simulink model "Samuno_Experimental"  (R2024b)
settings: Solver=ode4  StartTime=0.0  StopTime=Dur  FixedStep=simulation_ts  RelTol=1e-3  AbsTol=1e-3
InitFcn:
  | run("init_parts.m");
model workspace (MAT data in the model file):
  Control_Range_Lim = 0.2086
  D_Heading = 0
  I_Heading = 0
  P_Heading = 1
  control_ts = 0.4
  kd_pitch = 0
  kd_roll = 0.1
  kp_pitch = 4
  kp_roll = 4
  random_velocity = 0.72
  switch_val = 0.1032
values from neighbouring files (symbols this model uses):
  Nose = evalin('base', 'Nose')    [createSimulinkGUI.m]
  xCOB = xSliderCOB.Value    [createSimulinkGUI.m]
  zCOB = ySliderCOB.Value    [createSimulinkGUI.m]
undefined symbols (not defined in the file or in its folder): Caudal, colors, Force_Scale, gravity, Mid_Body, Mid_Fins, noise_mean, noise_sample_time, noise_var, Pect, Pedunc, TotalMass, X, Y, Z
libraries: nesl_utility x84, sm_lib x53
(part 3 of 3)

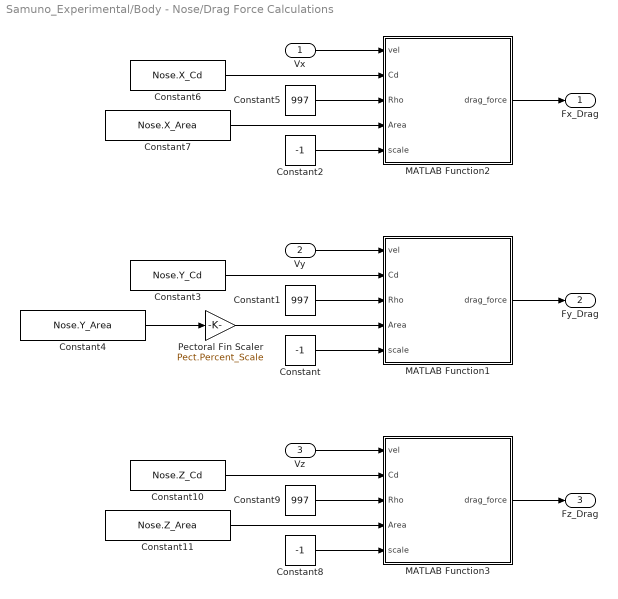
== system Samuno_Experimental/Body - Nose/Drag Force Calculations ==
  Vx : Inport
  Vy : Inport  Port=2
  Vz : Inport  Port=3
  Constant : Constant  Value=-1
  Constant1 : Constant  Value=997
  Constant10 : Constant  Value=Nose.Z_Cd
  Constant11 : Constant  Value=Nose.Z_Area
  Constant2 : Constant  Value=-1
  Constant3 : Constant  Value=Nose.Y_Cd
  Constant4 : Constant  Value=Nose.Y_Area
  Constant5 : Constant  Value=997
  Constant6 : Constant  Value=Nose.X_Cd
  Constant7 : Constant  Value=Nose.X_Area
  Constant8 : Constant  Value=-1
  Constant9 : Constant  Value=997
  MATLAB Function1 : MATLAB Function  TreatAsAtomicUnit=on
  MATLAB Function2 : MATLAB Function  TreatAsAtomicUnit=on
  MATLAB Function3 : MATLAB Function  TreatAsAtomicUnit=on
  Pectoral Fin Scaler : Gain  Gain=Pect.Percent_Scale
  Fx_Drag : Outport
  Fy_Drag : Outport  Port=2
  Fz_Drag : Outport  Port=3
  wires:
  Constant1/1 -> MATLAB Function1/3(Rho)
  MATLAB Function1/1(drag_force) -> Fy_Drag/1
  Constant4/1 -> Pectoral Fin Scaler/1
  Constant/1 -> MATLAB Function1/5(scale)
  Vy/1 -> MATLAB Function1/1(vel)
  Constant3/1 -> MATLAB Function1/2(Cd)
  Constant6/1 -> MATLAB Function2/2(Cd)
  Constant2/1 -> MATLAB Function2/5(scale)
  Constant7/1 -> MATLAB Function2/4(Area)
  Vx/1 -> MATLAB Function2/1(vel)
  MATLAB Function2/1(drag_force) -> Fx_Drag/1
  Constant5/1 -> MATLAB Function2/3(Rho)
  MATLAB Function3/1(drag_force) -> Fz_Drag/1
  Constant8/1 -> MATLAB Function3/5(scale)
  Constant11/1 -> MATLAB Function3/4(Area)
  Constant10/1 -> MATLAB Function3/2(Cd)
  Vz/1 -> MATLAB Function3/1(vel)
  Constant9/1 -> MATLAB Function3/3(Rho)
  Pectoral Fin Scaler/1 -> MATLAB Function1/4(Area)

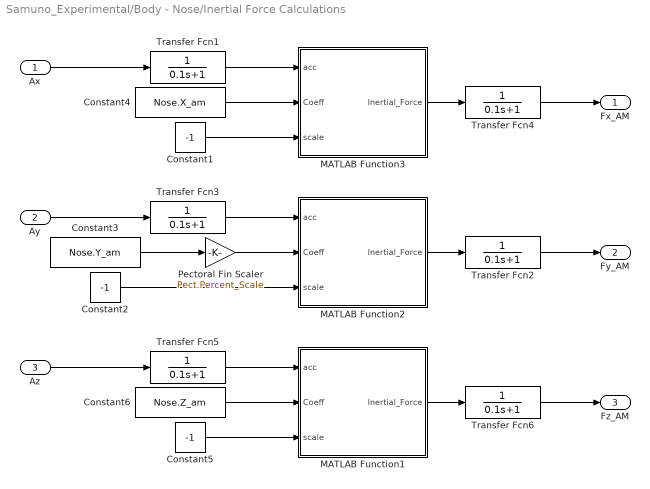
== system Samuno_Experimental/Body - Nose/Inertial Force Calculations ==
  Ax : Inport
  Ay : Inport  Port=2
  Az : Inport  Port=3
  Constant1 : Constant  Value=-1
  Constant2 : Constant  Value=-1
  Constant3 : Constant  Value=Nose.Y_am
  Constant4 : Constant  Value=Nose.X_am
  Constant5 : Constant  Value=-1
  Constant6 : Constant  Value=Nose.Z_am
  MATLAB Function1 : MATLAB Function  TreatAsAtomicUnit=on
  MATLAB Function2 : MATLAB Function  TreatAsAtomicUnit=on
  MATLAB Function3 : MATLAB Function  TreatAsAtomicUnit=on
  Pectoral Fin Scaler : Gain  Gain=Pect.Percent_Scale
  Transfer Fcn{1..6} (6 alike) : TransferFcn  Denominator=[0.1 1]
  Fx_AM : Outport
  Fy_AM : Outport  Port=2
  Fz_AM : Outport  Port=3
  wires:
  Ax/1 -> Transfer Fcn1/1
  Constant1/1 -> MATLAB Function3/3(scale)
  Transfer Fcn1/1 -> MATLAB Function3/1(acc)
  Constant4/1 -> MATLAB Function3/2(Coeff)
  Transfer Fcn4/1 -> Fx_AM/1
  MATLAB Function3/1(Inertial_Force) -> Transfer Fcn4/1
  Ay/1 -> Transfer Fcn3/1
  Constant2/1 -> MATLAB Function2/3(scale)
  Transfer Fcn3/1 -> MATLAB Function2/1(acc)
  Constant3/1 -> Pectoral Fin Scaler/1
  Transfer Fcn2/1 -> Fy_AM/1
  MATLAB Function2/1(Inertial_Force) -> Transfer Fcn2/1
  Az/1 -> Transfer Fcn5/1
  Constant5/1 -> MATLAB Function1/3(scale)
  Transfer Fcn5/1 -> MATLAB Function1/1(acc)
  Constant6/1 -> MATLAB Function1/2(Coeff)
  Transfer Fcn6/1 -> Fz_AM/1
  MATLAB Function1/1(Inertial_Force) -> Transfer Fcn6/1
  Pectoral Fin Scaler/1 -> MATLAB Function2/2(Coeff)

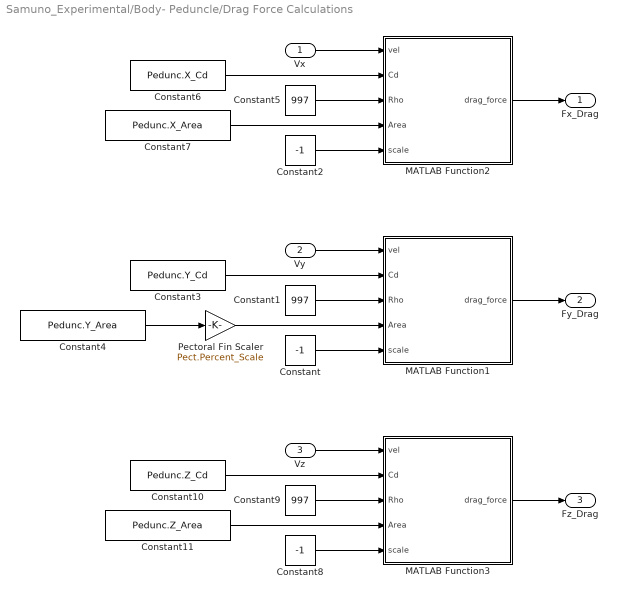
== system Samuno_Experimental/Body- Peduncle/Drag Force Calculations ==
  Vx : Inport
  Vy : Inport  Port=2
  Vz : Inport  Port=3
  Constant : Constant  Value=-1
  Constant1 : Constant  Value=997
  Constant10 : Constant  Value=Pedunc.Z_Cd
  Constant11 : Constant  Value=Pedunc.Z_Area
  Constant2 : Constant  Value=-1
  Constant3 : Constant  Value=Pedunc.Y_Cd
  Constant4 : Constant  Value=Pedunc.Y_Area
  Constant5 : Constant  Value=997
  Constant6 : Constant  Value=Pedunc.X_Cd
  Constant7 : Constant  Value=Pedunc.X_Area
  Constant8 : Constant  Value=-1
  Constant9 : Constant  Value=997
  MATLAB Function1 : MATLAB Function  TreatAsAtomicUnit=on
  MATLAB Function2 : MATLAB Function  TreatAsAtomicUnit=on
  MATLAB Function3 : MATLAB Function  TreatAsAtomicUnit=on
  Pectoral Fin Scaler : Gain  Gain=Pect.Percent_Scale
  Fx_Drag : Outport
  Fy_Drag : Outport  Port=2
  Fz_Drag : Outport  Port=3
  wires:
  Constant1/1 -> MATLAB Function1/3(Rho)
  MATLAB Function1/1(drag_force) -> Fy_Drag/1
  Constant4/1 -> Pectoral Fin Scaler/1
  Constant/1 -> MATLAB Function1/5(scale)
  Vy/1 -> MATLAB Function1/1(vel)
  Constant3/1 -> MATLAB Function1/2(Cd)
  Constant6/1 -> MATLAB Function2/2(Cd)
  Constant2/1 -> MATLAB Function2/5(scale)
  Constant7/1 -> MATLAB Function2/4(Area)
  Vx/1 -> MATLAB Function2/1(vel)
  MATLAB Function2/1(drag_force) -> Fx_Drag/1
  Constant5/1 -> MATLAB Function2/3(Rho)
  MATLAB Function3/1(drag_force) -> Fz_Drag/1
  Constant8/1 -> MATLAB Function3/5(scale)
  Constant11/1 -> MATLAB Function3/4(Area)
  Constant10/1 -> MATLAB Function3/2(Cd)
  Vz/1 -> MATLAB Function3/1(vel)
  Constant9/1 -> MATLAB Function3/3(Rho)
  Pectoral Fin Scaler/1 -> MATLAB Function1/4(Area)

== system Samuno_Experimental/Body- Peduncle/Inertial Force Calculations ==
  Ax : Inport
  Ay : Inport  Port=2
  Az : Inport  Port=3
  Constant1 : Constant  Value=-1
  Constant2 : Constant  Value=-1
  Constant3 : Constant  Value=Pedunc.Y_am
  Constant4 : Constant  Value=Pedunc.X_am
  Constant5 : Constant  Value=-1
  Constant6 : Constant  Value=Pedunc.Z_am
  MATLAB Function1 : MATLAB Function  TreatAsAtomicUnit=on
  MATLAB Function2 : MATLAB Function  TreatAsAtomicUnit=on
  MATLAB Function3 : MATLAB Function  TreatAsAtomicUnit=on
  Pectoral Fin Scaler : Gain  Gain=Pect.Percent_Scale
  Transfer Fcn1 : TransferFcn  Numerator=1.5  Denominator=[0.005 1]
  Transfer Fcn2 : TransferFcn  Numerator=1.5  Denominator=[0.005 1]
  Transfer Fcn3 : TransferFcn  Numerator=1.5  Denominator=[0.005 1]
  Fx_AM : Outport
  Fy_AM : Outport  Port=2
  Fz_AM : Outport  Port=3
  wires:
  Constant1/1 -> MATLAB Function3/3(scale)
  Ax/1 -> MATLAB Function3/1(acc)
  Constant4/1 -> MATLAB Function3/2(Coeff)
  Transfer Fcn1/1 -> Fx_AM/1
  MATLAB Function3/1(Inertial_Force) -> Transfer Fcn1/1
  Constant2/1 -> MATLAB Function2/3(scale)
  Ay/1 -> MATLAB Function2/1(acc)
  Constant3/1 -> Pectoral Fin Scaler/1
  Transfer Fcn2/1 -> Fy_AM/1
  MATLAB Function2/1(Inertial_Force) -> Transfer Fcn2/1
  Constant5/1 -> MATLAB Function1/3(scale)
  Az/1 -> MATLAB Function1/1(acc)
  Constant6/1 -> MATLAB Function1/2(Coeff)
  Transfer Fcn3/1 -> Fz_AM/1
  MATLAB Function1/1(Inertial_Force) -> Transfer Fcn3/1
  Pectoral Fin Scaler/1 -> MATLAB Function2/2(Coeff)

== system Samuno_Experimental/Caudal Fin/Drag Force Calculations ==
  vy : Inport
  Constant3 : Constant  Value=Caudal.Y_Area
  Constant5 : Constant  Value=-1
  Constant6 : Constant  Value=997
  Constant8 : Constant  Value=Caudal.Y_Cd
  MATLAB Function1 : MATLAB Function  TreatAsAtomicUnit=on
  Fy_Drag : Outport
  wires:
  MATLAB Function1/1(drag_force) -> Fy_Drag/1
  vy/1 -> MATLAB Function1/1(vel)
  Constant3/1 -> MATLAB Function1/4(Area)
  Constant6/1 -> MATLAB Function1/3(Rho)
  Constant8/1 -> MATLAB Function1/2(Cd)
  Constant5/1 -> MATLAB Function1/5(scale)

== system Samuno_Experimental/Caudal Fin/Inertial Force Calculations ==
  Ay : Inport
  Constant : Constant  Value=-1
  Constant3 : Constant  Value=Caudal.Y_am
  MATLAB Function1 : MATLAB Function  TreatAsAtomicUnit=on
  Transfer Fcn1 : TransferFcn  Numerator=1.5  Denominator=[0.005 1]
  Fy_AM : Outport
  wires:
  Constant3/1 -> MATLAB Function1/2(Coeff)
  MATLAB Function1/1(Inertial_Force) -> Transfer Fcn1/1
  Transfer Fcn1/1 -> Fy_AM/1
  Constant/1 -> MATLAB Function1/3(scale)
  Ay/1 -> MATLAB Function1/1(acc)

== system Samuno_Experimental/Dorsal-Anal Fins/Drag Force Calculations ==
  vy : Inport
  Constant3 : Constant  Value=Mid_Fins.Y_Cd
  Constant4 : Constant  Value=Mid_Fins.Y_Area
  Constant8 : Constant  Value=-1
  Constant9 : Constant  Value=997
  MATLAB Function1 : MATLAB Function  TreatAsAtomicUnit=on
  Fy_Drag : Outport
  wires:
  MATLAB Function1/1(drag_force) -> Fy_Drag/1
  Constant8/1 -> MATLAB Function1/5(scale)
  Constant9/1 -> MATLAB Function1/3(Rho)
  Constant4/1 -> MATLAB Function1/4(Area)
  Constant3/1 -> MATLAB Function1/2(Cd)
  vy/1 -> MATLAB Function1/1(vel)

== system Samuno_Experimental/Dorsal-Anal Fins/Drag Force Calculations1 ==
  vy : Inport
  Constant1 : Constant  Value=Mid_Fins.Y_Cd
  Constant3 : Constant  Value=997
  Constant4 : Constant  Value=Mid_Fins.Y_Area
  Constant8 : Constant  Value=-1
  MATLAB Function1 : MATLAB Function  TreatAsAtomicUnit=on
  Fy_Drag : Outport
  wires:
  vy/1 -> MATLAB Function1/1(vel)
  Constant4/1 -> MATLAB Function1/4(Area)
  MATLAB Function1/1(drag_force) -> Fy_Drag/1
  Constant1/1 -> MATLAB Function1/2(Cd)
  Constant3/1 -> MATLAB Function1/3(Rho)
  Constant8/1 -> MATLAB Function1/5(scale)

== system Samuno_Experimental/Dorsal-Anal Fins/Inertial Force Calculations ==
  Ay : Inport
  Constant : Constant  Value=-1
  Constant3 : Constant  Value=Mid_Fins.Y_am
  MATLAB Function1 : MATLAB Function  TreatAsAtomicUnit=on
  Transfer Fcn1 : TransferFcn  Numerator=1.5  Denominator=[0.005 1]
  Fy_AM : Outport
  wires:
  Constant3/1 -> MATLAB Function1/2(Coeff)
  MATLAB Function1/1(Inertial_Force) -> Transfer Fcn1/1
  Ay/1 -> MATLAB Function1/1(acc)
  Constant/1 -> MATLAB Function1/3(scale)
  Transfer Fcn1/1 -> Fy_AM/1

== system Samuno_Experimental/Dorsal-Anal Fins/Inertial Force Calculations1 ==
  Ay1 : Inport
  Constant : Constant  Value=-1
  Constant1 : Constant  Value=Mid_Fins.Y_am
  MATLAB Function2 : MATLAB Function  TreatAsAtomicUnit=on
  Transfer Fcn2 : TransferFcn  Numerator=1.5  Denominator=[0.005 1]
  Fy_AM1 : Outport
  wires:
  Transfer Fcn2/1 -> Fy_AM1/1
  Constant/1 -> MATLAB Function2/3(scale)
  MATLAB Function2/1(Inertial_Force) -> Transfer Fcn2/1
  Ay1/1 -> MATLAB Function2/1(acc)
  Constant1/1 -> MATLAB Function2/2(Coeff)

== system Samuno_Experimental/Left Pectoral/Drag Force Calculations ==
  Vz : Inport
  Constant1 : Constant  Value=Pect.Y_Cd
  Constant3 : Constant  Value=997
  Constant4 : Constant  Value=Pect.Y_Area
  Constant8 : Constant  Value=-1
  MATLAB Function1 : MATLAB Function  TreatAsAtomicUnit=on
  Fz_Drag : Outport
  wires:
  Constant1/1 -> MATLAB Function1/2(Cd)
  Constant3/1 -> MATLAB Function1/3(Rho)
  Constant8/1 -> MATLAB Function1/5(scale)
  Constant4/1 -> MATLAB Function1/4(Area)
  MATLAB Function1/1(drag_force) -> Fz_Drag/1
  Vz/1 -> MATLAB Function1/1(vel)

== system Samuno_Experimental/Left Pectoral/Inertial Force Calculations ==
  Az : Inport
  Constant : Constant  Value=-1
  Constant1 : Constant  Value=Pect.Y_am
  MATLAB Function2 : MATLAB Function  TreatAsAtomicUnit=on
  Transfer Fcn1 : TransferFcn  Denominator=[0.1 1]
  Transfer Fcn3 : TransferFcn  Denominator=[0.1 1]
  Fz_AM : Outport
  wires:
  MATLAB Function2/1(Inertial_Force) -> Transfer Fcn1/1
  Transfer Fcn1/1 -> Fz_AM/1
  Az/1 -> Transfer Fcn3/1
  Constant1/1 -> MATLAB Function2/2(Coeff)
  Transfer Fcn3/1 -> MATLAB Function2/1(acc)
  Constant/1 -> MATLAB Function2/3(scale)

== system Samuno_Experimental/Right Pectoral/Drag Force Calculations ==
  Vz : Inport
  Constant1 : Constant  Value=Pect.Y_Cd
  Constant3 : Constant  Value=997
  Constant4 : Constant  Value=Pect.Y_Area
  Constant8 : Constant  Value=-1
  MATLAB Function1 : MATLAB Function  TreatAsAtomicUnit=on
  Fz_Drag : Outport
  wires:
  Constant1/1 -> MATLAB Function1/2(Cd)
  Constant3/1 -> MATLAB Function1/3(Rho)
  Constant8/1 -> MATLAB Function1/5(scale)
  Constant4/1 -> MATLAB Function1/4(Area)
  MATLAB Function1/1(drag_force) -> Fz_Drag/1
  Vz/1 -> MATLAB Function1/1(vel)

== system Samuno_Experimental/Right Pectoral/Inertial Force Calculations ==
  Az : Inport
  Constant : Constant  Value=-1
  Constant1 : Constant  Value=Pect.Y_am
  MATLAB Function2 : MATLAB Function  TreatAsAtomicUnit=on
  Transfer Fcn1 : TransferFcn  Numerator=1.5  Denominator=[0.005 1]
  Fz_AM : Outport
  wires:
  MATLAB Function2/1(Inertial_Force) -> Transfer Fcn1/1
  Transfer Fcn1/1 -> Fz_AM/1
  Constant1/1 -> MATLAB Function2/2(Coeff)
  Az/1 -> MATLAB Function2/1(acc)
  Constant/1 -> MATLAB Function2/3(scale)

== matlab function Samuno_Experimental/Body - Middle/Drag Force Calculations/MATLAB Function3 ==
  data: vel input; drag_force output; Cd input; Rho input; Area input; scale input
function drag_force=Drag_Force(vel,Cd,Rho,Area,scale)

    drag_force=(1/2)*Rho*Cd*(Area)*(abs(vel)*vel)*scale;

end

== matlab function Samuno_Experimental/MATLAB Function ==
  data: matrix input; main_diag output
function main_diag = getDiagonals(matrix)
    % Check if the input is a 3x3 matrix
    if size(matrix, 1) ~= 3 || size(matrix, 2) ~= 3
        error('Input must be a 3x3 matrix');
    end

    % Extract the main diagonal
    main_diag = diag(matrix);
    
end

== matlab function Samuno_Experimental/Body - Middle/Inertial Force Calculations/MATLAB Function1 ==
  data: acc input; Inertial_Force output; Coeff input; scale input
function Inertial_Force=Added_Mass(acc,Coeff,scale)

    Inertial_Force=scale*acc*Coeff;

end

== matlab function Samuno_Experimental/Caudal Fin/Drag Force Calculations/MATLAB Function1 ==
  data: vel input; drag_force output; Cd input; Rho input; Area input; scale input
function drag_force=Drag_Force(vel,Cd,Rho,Area,scale)

    drag_force=(1/2)*Rho*Cd*(Area)*(abs(vel)*vel)*scale;

end

== matlab function Samuno_Experimental/Body - Middle/Inertial Force Calculations/MATLAB Function2 ==
  data: acc input; Inertial_Force output; Coeff input; scale input
function Inertial_Force=Added_Mass(acc,Coeff,scale)

    Inertial_Force=scale*acc*Coeff;

end

== matlab function Samuno_Experimental/Body - Middle/Inertial Force Calculations/MATLAB Function3 ==
  data: acc input; Inertial_Force output; Coeff input; scale input
function Inertial_Force=Added_Mass(acc,Coeff,scale)

    Inertial_Force=scale*acc*Coeff;

end

== matlab function Samuno_Experimental/Body - Nose/Drag Force Calculations/MATLAB Function2 ==
  data: vel input; drag_force output; Cd input; Rho input; Area input; scale input
function drag_force=Drag_Force(vel,Cd,Rho,Area,scale)

    drag_force=(1/2)*Rho*Cd*(Area)*(abs(vel)*vel)*scale;

end

== matlab function Samuno_Experimental/Body - Nose/Drag Force Calculations/MATLAB Function3 ==
  data: vel input; drag_force output; Cd input; Rho input; Area input; scale input
function drag_force=Drag_Force(vel,Cd,Rho,Area,scale)

    drag_force=(1/2)*Rho*Cd*(Area)*(abs(vel)*vel)*scale;

end

== matlab function Samuno_Experimental/Body - Nose/Inertial Force Calculations/MATLAB Function3 ==
  data: acc input; Inertial_Force output; Coeff input; scale input
function Inertial_Force=Added_Mass(acc,Coeff,scale)

    Inertial_Force=scale*acc*Coeff;

end

== matlab function Samuno_Experimental/Right Pectoral/Drag Force Calculations/MATLAB Function1 ==
  data: vel input; drag_force output; Cd input; Rho input; Area input; scale input
function drag_force=Drag_Force(vel,Cd,Rho,Area,scale)

    drag_force=(1/2)*Rho*Cd*(Area)*(abs(vel)*vel)*scale;

end

== matlab function Samuno_Experimental/Body- Peduncle/Drag Force Calculations/MATLAB Function3 ==
  data: vel input; drag_force output; Cd input; Rho input; Area input; scale input
function drag_force=Drag_Force(vel,Cd,Rho,Area,scale)

    drag_force=(1/2)*Rho*Cd*(Area)*(abs(vel)*vel)*scale;

end

== matlab function Samuno_Experimental/Body - Nose/Inertial Force Calculations/MATLAB Function2 ==
  data: acc input; Inertial_Force output; Coeff input; scale input
function Inertial_Force=Added_Mass(acc,Coeff,scale)

    Inertial_Force=scale*acc*Coeff;

end

== matlab function Samuno_Experimental/Body - Nose/Inertial Force Calculations/MATLAB Function1 ==
  data: acc input; Inertial_Force output; Coeff input; scale input
function Inertial_Force=Added_Mass(acc,Coeff,scale)

    Inertial_Force=scale*(acc)*Coeff;

end

== matlab function Samuno_Experimental/Dorsal-Anal Fins/Drag Force Calculations1/MATLAB Function1 ==
  data: vel input; drag_force output; Cd input; Rho input; Area input; scale input
function drag_force=Drag_Force(vel,Cd,Rho,Area,scale)

    drag_force=(1/2)*Rho*Cd*(Area)*(abs(vel)*vel)*scale;

end

== matlab function Samuno_Experimental/Left Pectoral/Drag Force Calculations/MATLAB Function1 ==
  data: vel input; drag_force output; Cd input; Rho input; Area input; scale input
function drag_force=Drag_Force(vel,Cd,Rho,Area,scale)

    drag_force=(1/2)*Rho*Cd*(Area)*(abs(vel)*vel)*scale;

end

== matlab function Samuno_Experimental/Left Pectoral/Inertial Force Calculations/MATLAB Function2 ==
  data: acc input; Inertial_Force output; Coeff input; scale input
function Inertial_Force=Added_Mass(acc,Coeff,scale)

    Inertial_Force=scale*acc*Coeff;

end

== matlab function Samuno_Experimental/Body- Peduncle/Inertial Force Calculations/MATLAB Function1 ==
  data: acc input; Inertial_Force output; Coeff input; scale input
function Inertial_Force=Added_Mass(acc,Coeff,scale)

    Inertial_Force=scale*(acc)*Coeff;

end

== matlab function Samuno_Experimental/Body- Peduncle/Inertial Force Calculations/MATLAB Function2 ==
  data: acc input; Inertial_Force output; Coeff input; scale input
function Inertial_Force=Added_Mass(acc,Coeff,scale)

    Inertial_Force=scale*acc*Coeff;

end

== matlab function Samuno_Experimental/Body- Peduncle/Inertial Force Calculations/MATLAB Function3 ==
  data: acc input; Inertial_Force output; Coeff input; scale input
function Inertial_Force=Added_Mass(acc,Coeff,scale)

    Inertial_Force=scale*acc*Coeff;

end

== matlab function Samuno_Experimental/Right Pectoral/Inertial Force Calculations/MATLAB Function2 ==
  data: acc input; Inertial_Force output; Coeff input; scale input
function Inertial_Force=Added_Mass(acc,Coeff,scale)

    Inertial_Force=scale*acc*Coeff;

end

== matlab function Samuno_Experimental/Dorsal-Anal Fins/Inertial Force Calculations/MATLAB Function1 ==
  data: acc input; Inertial_Force output; Coeff input; scale input
function Inertial_Force=Added_Mass(acc,Coeff,scale)

    Inertial_Force=scale*acc*Coeff;

end

== matlab function Samuno_Experimental/Caudal Fin/Inertial Force Calculations/MATLAB Function1 ==
  data: acc input; Inertial_Force output; Coeff input; scale input
function Inertial_Force=Added_Mass(acc,Coeff,scale)

    Inertial_Force=scale*acc*Coeff;

end

== matlab function Samuno_Experimental/Body- Peduncle/Drag Force Calculations/MATLAB Function1 ==
  data: vel input; drag_force output; Cd input; Rho input; Area input; scale input
function drag_force=Drag_Force(vel,Cd,Rho,Area,scale)

    drag_force=(1/2)*Rho*Cd*(Area)*(abs(vel)*vel)*scale;

end

== matlab function Samuno_Experimental/Body- Peduncle/Drag Force Calculations/MATLAB Function2 ==
  data: vel input; drag_force output; Cd input; Rho input; Area input; scale input
function drag_force=Drag_Force(vel,Cd,Rho,Area,scale)

    drag_force=(1/2)*Rho*Cd*(Area)*(abs(vel)*vel)*scale;

end

== matlab function Samuno_Experimental/Body - Middle/Drag Force Calculations/MATLAB Function1 ==
  data: vel input; drag_force output; Cd input; Rho input; Area input; scale input
function drag_force=Drag_Force(vel,Cd,Rho,Area,scale)

    drag_force=(1/2)*Rho*Cd*(Area)*(abs(vel)*vel)*scale;

end

== matlab function Samuno_Experimental/Body - Middle/Drag Force Calculations/MATLAB Function2 ==
  data: vel input; drag_force output; Cd input; Rho input; Area input; scale input
function drag_force=Drag_Force(vel,Cd,Rho,Area,scale)

    drag_force=(1/2)*Rho*Cd*(Area)*(abs(vel)*vel)*scale;

end

== matlab function Samuno_Experimental/Body - Nose/Drag Force Calculations/MATLAB Function1 ==
  data: vel input; drag_force output; Cd input; Rho input; Area input; scale input
function drag_force=Drag_Force(vel,Cd,Rho,Area,scale)

    drag_force=(1/2)*Rho*Cd*(Area)*(abs(vel)*vel)*scale;

end

== matlab function Samuno_Experimental/Dorsal-Anal Fins/Inertial Force Calculations1/MATLAB Function2 ==
  data: acc input; Inertial_Force output; Coeff input; scale input
function Inertial_Force=Added_Mass(acc,Coeff,scale)

    Inertial_Force=scale*acc*Coeff;

end

== matlab function Samuno_Experimental/Dorsal-Anal Fins/Drag Force Calculations/MATLAB Function1 ==
  data: vel input; drag_force output; Cd input; Rho input; Area input; scale input
function drag_force=Drag_Force(vel,Cd,Rho,Area,scale)

    drag_force=(1/2)*Rho*Cd*(Area)*(abs(vel)*vel)*scale;

end
